simulink model "Ex1_ON_OFF_Control"  (R2023b)
settings: Solver=FixedStepDiscrete  StartTime=0.0  StopTime=inf  FixedStep=0.1  RelTol=1e-3  EnableMultiTasking=on
libraries: arduinolib x1, arduinosensorlib x1
settings Model: ExtModeTrigDuration=2  Creator=Alejandro  LastModifiedBy=Alejandro
settings OptimizationCC: EnhancedBackFolding=on  PassReuseOutputArgsAs=Individual arguments  ZeroExternalMemoryAtStartup=off  ZeroInternalMemoryAtStartup=off  MaxStackSize=64  OptimizeBlockOrder=speed  DifferentSizesBufferReuse=on  OptimizationCustomize=off  EfficientTunableParamExpr=on
settings DebuggingCC: ParameterTunabilityLossMsg=error
settings HardwareCC: ProdBitPerInt=16  ProdBitPerPointer=16  ProdBitPerSizeT=16  ProdBitPerPtrDiffT=16  ProdLargestAtomicFloat=None  ProdWordSize=8  ProdHWDeviceType=Atmel->AVR
settings SFSimCC: MATLABDynamicMemAlloc=off
settings RTWCC: Description=Embedded Coder  SystemTargetFile=ert.tlc  HardwareBoard=Arduino Uno  TemplateMakefile=ert_default_tmf  Toolchain=Arduino AVR  BuildConfiguration=Faster Runs
settings CodeAppCC: ForceParamTrailComments=on  IgnoreCustomStorageClasses=off  OperatorAnnotations=on  SimulinkDataObjDesc=on  SFDataObjDesc=on  InsertBlockDesc=on
settings ERTTargetCC: SupportContinuousTime=on  SupportVariableSizeSignals=on  ExtModeTransport=3  ExtModeStaticAlloc=on  ExtModeAutomaticAllocSize=off  ExtModeStaticAllocSize=250  ExtModeMexFile=ext_xcp  ExtModeIntrfLevel=Level2 - Open

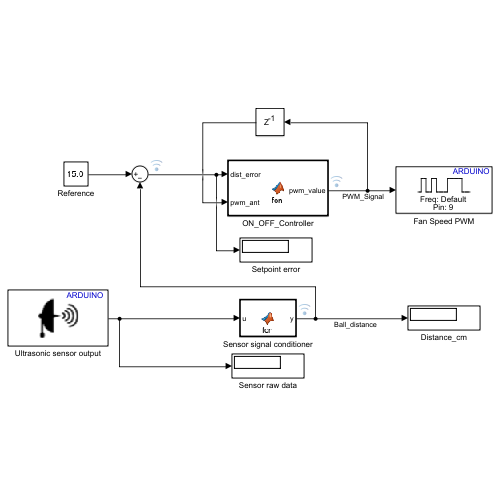
[thumbnail: Simulink's stored preview of the top-level diagram]
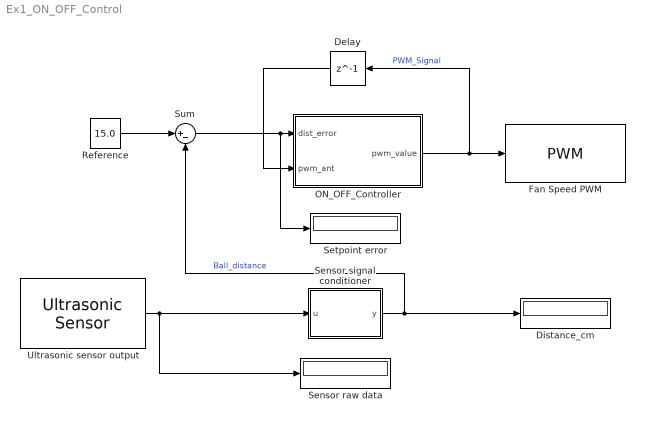
== system Ex1_ON_OFF_Control ==
  Delay : Delay  DelayLength=1
  Distance_cm : Display
  Fan Speed PWM : arduinolib/PWM  pinNumber=9  frequencyType=Default  desiredFrequency=490.2  achievableFrequency=490.2
  ON_OFF_Controller : MATLAB Function  TreatAsAtomicUnit=on
  Reference : Constant  Value=15.0
  Sensor raw data : Display
  Sensor signal conditioner : MATLAB Function  TreatAsAtomicUnit=on
  Setpoint error : Display
  Sum : Sum  Inputs=|+-
  Ultrasonic sensor output : arduinosensorlib/Ultrasonic Sensor  NumSignalPins=2  TrigPin=12  EchoPin=11  SignalPin=3  SampleTime_=0.1  blockPlatform=ARDUINO
  wires:
  Ultrasonic sensor output/1 -> Sensor signal conditioner/1(u), Sensor raw data/1
  Sensor signal conditioner/1(y) -> Distance_cm/1, Sum/2  "Ball_distance"
  Reference/1 -> Sum/1
  Sum/1 -> Setpoint error/1, ON_OFF_Controller/1(dist_error)
  ON_OFF_Controller/1(pwm_value) -> Delay/1, Fan Speed PWM/1  "PWM_Signal"
  Delay/1 -> ON_OFF_Controller/2(pwm_ant)

== matlab function Ex1_ON_OFF_Control/Sensor signal conditioner ==
  data: u input; y output
function y = fcn(u)

MAX_DIST = 30;

y=MAX_DIST-(u*100);

== matlab function Ex1_ON_OFF_Control/ON_OFF_Controller ==
  data: pwm_value output; dist_error input; pwm_ant input
function pwm_value = fcn(dist_error,pwm_ant)

HYSTERESYS_STEP=2.0;
OFF_MODE=82;
ON_MODE=182;
pwm_value=0;

% Set the OFF mode if it is over the given setpoint
if (dist_error >= HYSTERESYS_STEP)
    pwm_value=ON_MODE;
% Set the ON mode if it is below the given setpoint
elseif (dist_error <= -HYSTERESYS_STEP)
    pwm_value=OFF_MODE;
else
    pwm_value=pwm_ant;
end
